simulink model "bpskcanal"  (R2015a)
settings: Solver=ode45  StartTime=0.0  StopTime=10.0  RelTol=1e-3
libraries: commdigbbndpm3 x2, commchan3 x1, commrandsrc2 x1
settings Model: Creator=francisco  LastModifiedBy=francisco

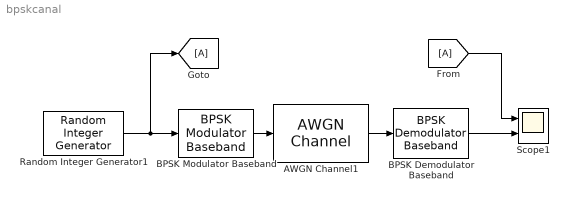
== system bpskcanal ==
  AWGN Channel1 : commchan3/AWGN Channel  InputProcessing=Columns as channels (frame based)  seed=67  noiseMode="Signal to noise ratio  (Eb/No)"  EbNodB=EbNo  EsNodB=10  SNRdB=10  bitsPerSym=1  Ps=1  Tsym=1  variance=1
  BPSK Demodulator Baseband : commdigbbndpm3/BPSK Demodulator Baseband  Ph=0  DecType=Hard decision  VarSource=Dialog  Variance=1  outDtype=Inherit via internal rule  derotateFactorWordLen=16
  BPSK Modulator Baseband : commdigbbndpm3/BPSK Modulator Baseband  Ph=0  outDtype=double  outWordLen=16  outUDDataType=sfix(16)  outFracLenMode=Best precision  outFracLen=15
  Random Integer Generator1 : commrandsrc2/Random Integer Generator  RequirementInfo={} %GIDa_a449ad49_6728_43c7_bd47_483ea2b92e0a  mul=2  seed=37  Ts=1  frameBased=off  sampPerFrame=1  orient=off  outDataType=double
  Scope1 : Scope  NumInputPorts=2
      settings: YMin=-5~-5  YMax=5~5  SaveName=ScopeData2  Decimation=100
  wires:
  Random Integer Generator1/1 -> [A], BPSK Modulator Baseband/1
  BPSK Modulator Baseband/1 -> AWGN Channel1/1
  AWGN Channel1/1 -> BPSK Demodulator Baseband/1
  [A] -> Scope1/1
  BPSK Demodulator Baseband/1 -> Scope1/2
